simulink library "lib_DriverRequests"  (R2017a)
settings: Solver=VariableStepAuto  StartTime=0.0  StopTime=10.0  RelTol=1e-3
undefined symbols (not defined in the file): cal, eng
libraries: simulink x9, EC2_libraries x1
settings Model: Creator=Di Russo  LastModifiedBy=Vraj M

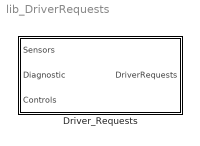
== system lib_DriverRequests ==
  Driver_Requests : Subsystem  RequirementInfo="{'other' 'HCU_Requirements.xlsx' '@Simulink_requirement_item_5' 'true' 'Determines the  driver''s intention i.e. status of the vehicle start, HCU on/off status and the Driver Intend Axle Torque from the sensor inputs.' '' } %GIDa_c835b258_06dc_4801_8a9e_97f7e56cbdd0"

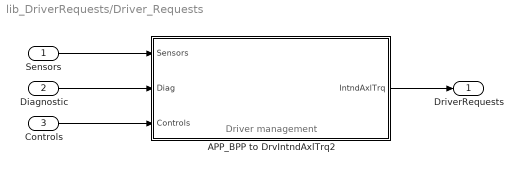
== system lib_DriverRequests/Driver_Requests ==
  note: Driver management
  Sensors : Inport
  "Diagnostic " : Inport  Port=2
  "Controls " : Inport  Port=3
  APP_BPP to DrvIntndAxlTrq2 : Subsystem
  DriverRequests : Outport
  wires:
  "Controls "/1 -> APP_BPP to DrvIntndAxlTrq2/3(Controls)
  "Diagnostic "/1 -> APP_BPP to DrvIntndAxlTrq2/2(Diag)
  APP_BPP to DrvIntndAxlTrq2/1(IntndAxlTrq) -> DriverRequests/1
  Sensors/1 -> APP_BPP to DrvIntndAxlTrq2/1(Sensors)

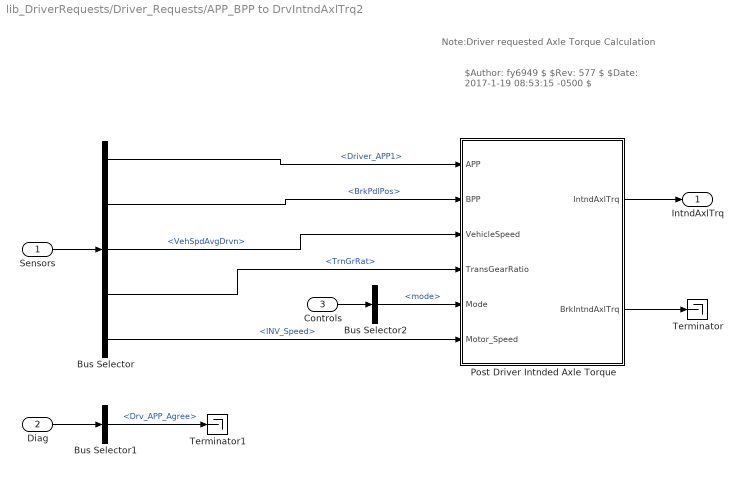
== system lib_DriverRequests/Driver_Requests/APP_BPP to DrvIntndAxlTrq2 ==
  note: $Author: fy6949 $
      | $Rev: 577 $
      | $Date: 2017-1-19 08:53:15 -0500  $
  note: Note:Driver requested Axle Torque Calculation
  Sensors : Inport
  Diag : Inport  Port=2
  Controls : Inport  Port=3
  Bus Selector : BusSelector  OutputSignals=from_Analog.Driver_APP1,from_CAN.fromVEH_CAN.from_BCM.BrkPdlPos,from_CAN.fromEBCAN.from_ECM.VehSpdAvgDrvn,from_CAN.fromVEH_CAN.from_TCM.TrnGrRat,from_CAN.fromHV_CAN.from_MCU.INV_VCU_01.INV_Speed
  Bus Selector1 : BusSelector  OutputSignals=CompSig.RawSig.Driver_SigDiag.Drv_APP_Agree
  Bus Selector2 : BusSelector  OutputSignals=mode
  Post Driver Intnded Axle Torque : Subsystem
  Terminator : Terminator
  Terminator1 : Terminator
  IntndAxlTrq : Outport
  wires:
  Bus Selector2/1 -> Post Driver Intnded Axle Torque/5(Mode)  "<mode>"
  Bus Selector1/1 -> Terminator1/1  "<Drv_APP_Agree>"
  Diag/1 -> Bus Selector1/1
  Post Driver Intnded Axle Torque/2(BrkIntndAxlTrq) -> Terminator/1
  Bus Selector/1 -> Post Driver Intnded Axle Torque/1(APP)  "<Driver_APP1>"
  Bus Selector/4 -> Post Driver Intnded Axle Torque/4(TransGearRatio)  "<TrnGrRat>"
  Bus Selector/5 -> Post Driver Intnded Axle Torque/6(Motor_Speed)  "<INV_Speed>"
  Bus Selector/3 -> Post Driver Intnded Axle Torque/3(VehicleSpeed)  "<VehSpdAvgDrvn>"
  Bus Selector/2 -> Post Driver Intnded Axle Torque/2(BPP)  "<BrkPdlPos>"
  Post Driver Intnded Axle Torque/1(IntndAxlTrq) -> IntndAxlTrq/1
  Controls/1 -> Bus Selector2/1
  Sensors/1 -> Bus Selector/1

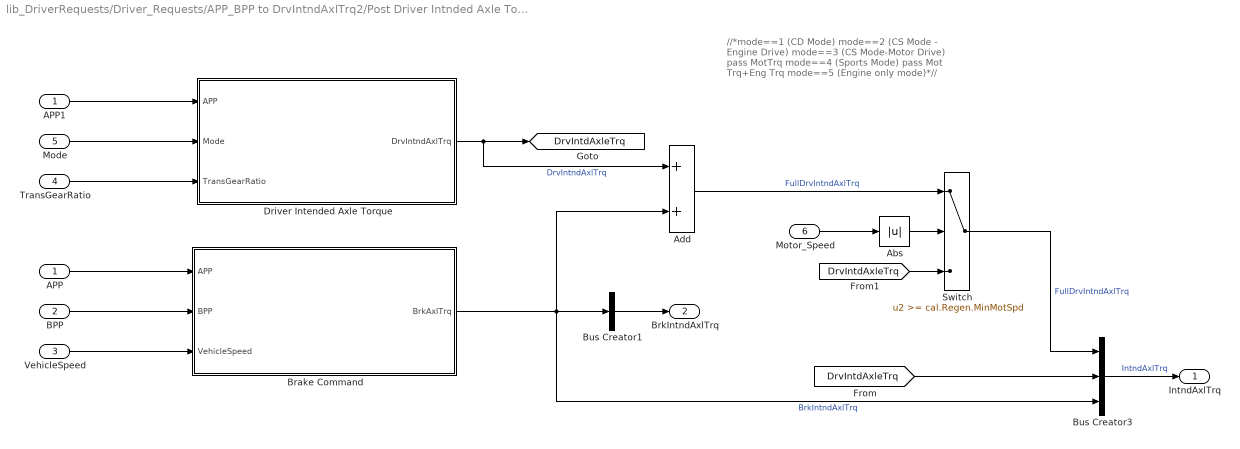
== system lib_DriverRequests/Driver_Requests/APP_BPP to DrvIntndAxlTrq2/Post Driver Intnded Axle Torque ==
  note: //*mode==1 (CD Mode)
      | mode==2 (CS Mode - Engine Drive)
      | mode==3 (CS Mode-Motor Drive) pass MotTrq
      | mode==4 (Sports Mode) pass Mot Trq+Eng Trq
      | mode==5 (Engine only mode)*//
  APP : Inport
  BPP : Inport  Port=2
  VehicleSpeed : Inport  Port=3
  TransGearRatio : Inport  Port=4
  Mode : Inport  Port=5
  Motor_Speed : Inport  Port=6
  APP1 : InportShadow
  Abs : Abs
  Add : Sum
  Brake Command : Subsystem
  Bus Creator1 : BusCreator  Inputs=1
  Bus Creator3 : BusCreator  Inputs=3
  Driver Intended Axle Torque : Subsystem
  Switch : Switch  Threshold=cal.Regen.MinMotSpd
  IntndAxlTrq : Outport
  BrkIntndAxlTrq : Outport  Port=2
  tag scope: DrvIntdAxleTrq=global
  wires:
  [DrvIntdAxleTrq] -> Switch/3
  APP1/1 -> Driver Intended Axle Torque/1(APP)
  [DrvIntdAxleTrq] -> Bus Creator3/2
  Bus Creator3/1 -> IntndAxlTrq/1  "IntndAxlTrq"
  Switch/1 -> Bus Creator3/1  "FullDrvIntndAxlTrq"
  Add/1 -> Switch/1  "FullDrvIntndAxlTrq"
  Abs/1 -> Switch/2
  Motor_Speed/1 -> Abs/1
  Bus Creator1/1 -> BrkIntndAxlTrq/1
  Brake Command/1(BrkAxlTrq) -> Bus Creator3/3, Bus Creator1/1, Add/2  "BrkIntndAxlTrq"
  TransGearRatio/1 -> Driver Intended Axle Torque/3(TransGearRatio)
  Mode/1 -> Driver Intended Axle Torque/2(Mode)
  VehicleSpeed/1 -> Brake Command/3(VehicleSpeed)
  BPP/1 -> Brake Command/2(BPP)
  Driver Intended Axle Torque/1(DrvIntndAxlTrq) -> [DrvIntdAxleTrq], Add/1  "DrvIntndAxlTrq"
  APP/1 -> Brake Command/1(APP)

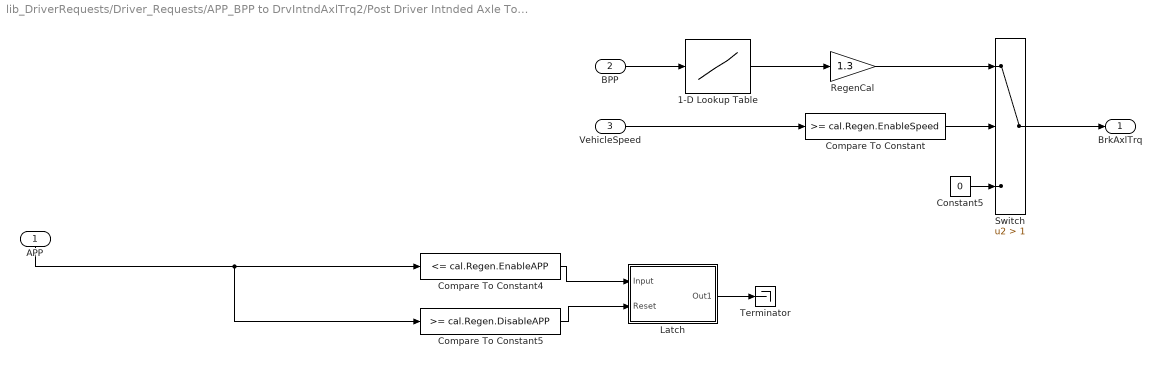
== system lib_DriverRequests/Driver_Requests/APP_BPP to DrvIntndAxlTrq2/Post Driver Intnded Axle Torque/Brake Command ==
  APP : Inport
  BPP : Inport  Port=2
  VehicleSpeed : Inport  Port=3
  1-D Lookup Table : Lookup_n-D  NumberOfTableDimensions=1  BreakpointsForDimension1=cal.Regen.BrakeAxleTrq.idx1_BrkPdlPos  Table=cal.Regen.BrakeAxleTrq.map  InternalRulePriority=Speed  RndMeth=Simplest  InputSameDT=on
  Compare To Constant : simulink/Logic and Bit Operations/Compare To Constant  relop=>=  const=cal.Regen.EnableSpeed  OutDataTypeStr=boolean
  Compare To Constant4 : simulink/Logic and Bit Operations/Compare To Constant  relop=<=  const=cal.Regen.EnableAPP  OutDataTypeStr=boolean
  Compare To Constant5 : simulink/Logic and Bit Operations/Compare To Constant  relop=>=  const=cal.Regen.DisableAPP  OutDataTypeStr=boolean
  Constant5 : Constant  Value=0
  Latch : Subsystem
  RegenCal : Gain  Gain=1.3
  Switch : Switch  Criteria=u2 > Threshold  Threshold=1
  Terminator : Terminator
  BrkAxlTrq : Outport
  wires:
  RegenCal/1 -> Switch/1
  Latch/1(Out1) -> Terminator/1
  Compare To Constant4/1 -> Latch/1(Input)
  Compare To Constant5/1 -> Latch/2(Reset)
  Constant5/1 -> Switch/3
  Compare To Constant/1 -> Switch/2
  BPP/1 -> 1-D Lookup Table/1
  APP/1 -> Compare To Constant4/1, Compare To Constant5/1
  Switch/1 -> BrkAxlTrq/1
  1-D Lookup Table/1 -> RegenCal/1
  VehicleSpeed/1 -> Compare To Constant/1

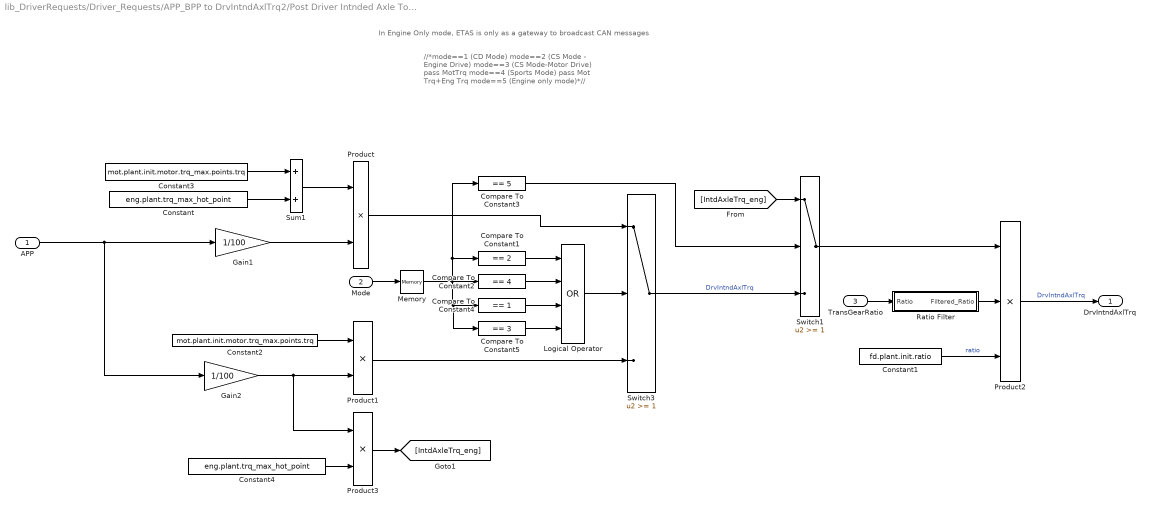
== system lib_DriverRequests/Driver_Requests/APP_BPP to DrvIntndAxlTrq2/Post Driver Intnded Axle Torque/Driver Intended Axle Torque ==
  note: //*mode==1 (CD Mode)
      | mode==2 (CS Mode - Engine Drive)
      | mode==3 (CS Mode-Motor Drive) pass MotTrq
      | mode==4 (Sports Mode) pass Mot Trq+Eng Trq
      | mode==5 (Engine only mode)*//
  note: In Engine Only mode, ETAS is only as a gateway to broadcast CAN messages
  APP : Inport
  Mode : Inport  Port=2
  TransGearRatio : Inport  Port=3
  Compare To Constant1 : simulink/Logic and Bit Operations/Compare To Constant  relop===  const=2  OutDataTypeStr=boolean
  Compare To Constant2 : simulink/Logic and Bit Operations/Compare To Constant  relop===  const=4  OutDataTypeStr=boolean
  Compare To Constant3 : simulink/Logic and Bit Operations/Compare To Constant  relop===  const=5  OutDataTypeStr=boolean
  Compare To Constant4 : simulink/Logic and Bit Operations/Compare To Constant  relop===  const=1  OutDataTypeStr=boolean
  Compare To Constant5 : simulink/Logic and Bit Operations/Compare To Constant  relop===  const=3  OutDataTypeStr=boolean
  Constant : Constant  Value=eng.plant.trq_max_hot_point  VectorParams1D=off
  Constant1 : Constant  Value=fd.plant.init.ratio
  Constant2 : Constant  Value=mot.plant.init.motor.trq_max.points.trq  VectorParams1D=off
  Constant3 : Constant  Value=mot.plant.init.motor.trq_max.points.trq  VectorParams1D=off
  Constant4 : Constant  Value=eng.plant.trq_max_hot_point  VectorParams1D=off
  Gain1 : Gain  Gain=1/100
  Gain2 : Gain  Gain=1/100
  Logical Operator : Logic  Operator=OR  Inputs=4  AllPortsSameDT=off  OutDataTypeStr=boolean
  Memory : Memory
  Product : Product  RndMeth=Zero
  Product1 : Product  RndMeth=Zero
  Product2 : Product  Inputs=3  RndMeth=Zero
  Product3 : Product  RndMeth=Zero
  Ratio Filter : Subsystem
  Sum1 : Sum
  Switch1 : Switch  Threshold=1
  Switch3 : Switch  Threshold=1
  DrvIntndAxlTrq : Outport
  wires:
  Compare To Constant5/1 -> Logical Operator/4
  Compare To Constant4/1 -> Logical Operator/3
  APP/1 -> Gain1/1, Gain2/1
  Switch1/1 -> Product2/1
  [IntdAxleTrq_eng] -> Switch1/1
  Logical Operator/1 -> Switch3/2
  Constant4/1 -> Product3/2
  Compare To Constant3/1 -> Switch1/2
  Product3/1 -> [IntdAxleTrq_eng]
  Switch3/1 -> Switch1/3  "DrvIntndAxlTrq"
  Constant/1 -> Sum1/2
  Compare To Constant2/1 -> Logical Operator/2
  Sum1/1 -> Product/1
  Compare To Constant1/1 -> Logical Operator/1
  Constant3/1 -> Sum1/1
  Memory/1 -> Compare To Constant1/1, Compare To Constant3/1, Compare To Constant2/1, Compare To Constant4/1, Compare To Constant5/1
  Gain1/1 -> Product/2
  Product2/1 -> DrvIntndAxlTrq/1  "DrvIntndAxlTrq"
  TransGearRatio/1 -> Ratio Filter/1(Ratio)
  Product1/1 -> Switch3/3
  Constant1/1 -> Product2/3  "ratio"
  Mode/1 -> Memory/1
  Product/1 -> Switch3/1
  Gain2/1 -> Product3/1, Product1/2
  Ratio Filter/1(Filtered_Ratio) -> Product2/2
  Constant2/1 -> Product1/1

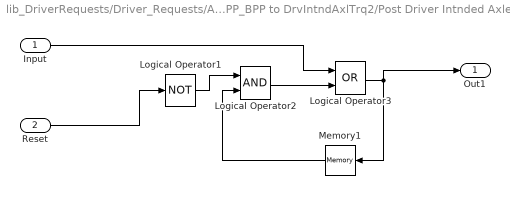
== system lib_DriverRequests/Driver_Requests/APP_BPP to DrvIntndAxlTrq2/Post Driver Intnded Axle Torque/Brake Command/Latch ==
  Input : Inport
  Reset : Inport  Port=2
  Logical Operator1 : Logic  Operator=NOT  AllPortsSameDT=off  OutDataTypeStr=boolean
  Logical Operator2 : Logic  AllPortsSameDT=off  OutDataTypeStr=boolean
  Logical Operator3 : Logic  Operator=OR  AllPortsSameDT=off  OutDataTypeStr=boolean
  Memory1 : Memory
  Out1 : Outport
  wires:
  Input/1 -> Logical Operator3/1
  Logical Operator1/1 -> Logical Operator2/1
  Logical Operator3/1 -> Memory1/1, Out1/1
  Memory1/1 -> Logical Operator2/2
  Reset/1 -> Logical Operator1/1
  Logical Operator2/1 -> Logical Operator3/2

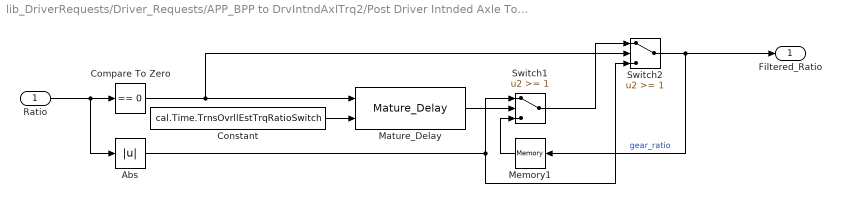
== system lib_DriverRequests/Driver_Requests/APP_BPP to DrvIntndAxlTrq2/Post Driver Intnded Axle Torque/Driver Intended Axle Torque/Ratio Filter ==
  Ratio : Inport
  Abs : Abs
  Compare To Zero : simulink/Logic and Bit Operations/Compare To Zero  relop===  OutDataTypeStr=boolean
  Constant : Constant  Value=cal.Time.TrnsOvrllEstTrqRatioSwitch
  Mature_Delay : EC2_libraries/Mature_Delay
  Memory1 : Memory  X0=1
  Switch1 : Switch  Threshold=1
  Switch2 : Switch  Threshold=1
  Filtered_Ratio : Outport
  wires:
  Switch2/1 -> Memory1/1, Filtered_Ratio/1  "gear_ratio"
  Memory1/1 -> Switch1/3
  Mature_Delay/1 -> Switch1/2
  Constant/1 -> Mature_Delay/2
  Switch1/1 -> Switch2/1
  Abs/1 -> Switch2/3, Switch1/1
  Compare To Zero/1 -> Switch2/2, Mature_Delay/1
  Ratio/1 -> Abs/1, Compare To Zero/1
